simulink model "WDS_with_AttackDetection"  (R2021a)
settings: Solver=FixedStepDiscrete  StartTime=0.0  StopTime=T_final  FixedStep=T_sample  RelTol=1e-3
values from neighbouring files (symbols this model uses):
  A_bar_d = readmatrix('A_bar_d.csv')    [Run_model_with_attackDetection.m]
  attack_tank_full = zeros(size(attack_tank,1),n_meas)    [Run_results.m]    (also in Run_results_new.m; time_domain_sim.m)
  b1_1 = readmatrix(append(datapath,'MLP1\b1.csv'))    [Run_model_with_attackDetection.m]
  b1_2 = readmatrix(append(datapath,'MLP2\b1.csv'))    [Run_model_with_attackDetection.m]
  b2_1 = readmatrix(append(datapath,'MLP1\b2.csv'))    [Run_model_with_attackDetection.m]
  b2_2 = readmatrix(append(datapath,'MLP2\b2.csv'))    [Run_model_with_attackDetection.m]
  b3_1 = readmatrix(append(datapath,'MLP1\b3.csv'))    [Run_model_with_attackDetection.m]
  b3_2 = readmatrix(append(datapath,'MLP2\b3.csv'))    [Run_model_with_attackDetection.m]
  b4_1 = readmatrix(append(datapath,'MLP1\b4.csv'))    [Run_model_with_attackDetection.m]
  b4_2 = readmatrix(append(datapath,'MLP2\b4.csv'))    [Run_model_with_attackDetection.m]
  B_bar_d = readmatrix('B_bar_d.csv')    [Run_model_with_attackDetection.m]
  C_obsv_d = readmatrix('C_obsv_d.csv')    [Run_model_with_attackDetection.m]
  Cm = ones(1,n_states)    [Run_model_with_attackDetection.m]
  D_obsv_d = readmatrix('D_obsv_d.csv')    [Run_model_with_attackDetection.m]
  E0_full = zeros(T,n_meas)    [Run_results.m]    (also in Run_results_new.m; time_domain_sim.m)
  eta = 0.7    [Run_model_with_attackDetection.m]
  H0_perp_full = eye(size(H0_full,1)) - H0_full*H0_full_pinv    [Run_model_with_attackDetection.m]
  I_attack_local = I_attack(1:n_attack)    [Run_results.m]    (also in Run_results_new.m; time_domain_sim.m)
  K = place(A_bar_d,B_bar_d,Pc)    [Run_model_with_attackDetection.m]
  k0 = 42    [Run_model_with_attackDetection.m]
  Lu = F-A_bar_d.'*H0_full_pinv*H1_full    [Run_model_with_attackDetection.m]
  Ly = A_bar_d.'*H0_full_pinv    [Run_model_with_attackDetection.m]
  M1 = readmatrix('M1.csv')    [Run_model_with_attackDetection.m]
  M2 = readmatrix('M2.csv')    [Run_model_with_attackDetection.m]
  n_meas = size(C_obsv_d,1)    [Run_model_with_attackDetection.m]
  offset = -inv(B_bar_d)*(A_bar_d-eye(n_states))*xd    [Run_model_with_attackDetection.m]
  p_MLP1 = load('P1.mat').P1    [Run_model_with_attackDetection.m]
  p_MLP2 = load('P2.mat').P2    [Run_model_with_attackDetection.m]
  Q0 = ones(n_meas,T)    [Run_model_with_attackDetection.m]
  T = 8    [Run_model_with_attackDetection.m]    (also in align_attack_dataset.m)
  T_sample = 0.01    [Run_model_with_attackDetection.m]
  T_start_attack = 0.1*T_final    (= 0.8)    [Run_model_with_attackDetection.m]
  T_start_detect = T_start_attack+T*T_sample    (= 0.88)    [Run_model_with_attackDetection.m]
  tau2 = readmatrix('tau2.csv')    [Run_model_with_attackDetection.m]
  U0 = zeros(n_int,T+1)    [Run_model_with_attackDetection.m]
  w1_1 = readmatrix(append(datapath,'\MLP1\w1.csv'))    [Run_model_with_attackDetection.m]
  w1_2 = readmatrix(append(datapath,'\MLP2\w1.csv'))    [Run_model_with_attackDetection.m]
  w2_1 = readmatrix(append(datapath,'MLP1\w2.csv'))    [Run_model_with_attackDetection.m]
  w2_2 = readmatrix(append(datapath,'MLP2\w2.csv'))    [Run_model_with_attackDetection.m]
  w3_1 = readmatrix(append(datapath,'MLP1\w3.csv'))    [Run_model_with_attackDetection.m]
  w3_2 = readmatrix(append(datapath,'MLP2\w3.csv'))    [Run_model_with_attackDetection.m]
  w4_1 = readmatrix(append(datapath,'MLP1\w4.csv'))    [Run_model_with_attackDetection.m]
  w4_2 = readmatrix(append(datapath,'MLP2\w4.csv'))    [Run_model_with_attackDetection.m]
  x0 = 0.3+ 0.2*rand(n_states,1)    [Run_model_with_attackDetection.m]
  xd = 0.5*ones(n_states,1)    [Run_model_with_attackDetection.m]
  Y0 = zeros(n_meas,T)    [Run_model_with_attackDetection.m]
undefined symbols (not defined in the file or in its folder): F, H0_full, H1_full, n_int, n_states, T_start_opt
libraries: simulink x15
(part 2 of 2)

== matlab function WDS_with_AttackDetection/False Data Injection Attacks3/sample_based Moving-horizon FDIA ==
  data: E output; e output double; et input; attack_tank_full parameter; M1 parameter; M2 parameter; tau2 parameter; T parameter
function [E,e] = fcn(et, attack_tank_full, M1, M2,tau2,T)
%% function [E,e] = fcn(et, attack_tank_full, M1, M2,tau2)
% sample-based moving horizon FDIA
% optimization problem or returns zeros if infeasible:
%         Maximize: ||M1*[e_history; e_i]||_2 
%         Subject to: ||M2*[e_history; e_i||_2 <= tau
%                      e_i \in e_data
% Inputs: 
%         - et [n_meas-by-T]         : cahce
%         - attack_tank_full [N_data-by-n_meas]: tank of pre-generated attacks
%         - M1 [n_m1-by-(T*n_meas)]  : Attack impact operator
%         - M2 [n_m2-by-(T*n_meas)]  : Detection residual operator
%         - tau2 [scalar]            : Detection threshold
% Output:
%         - E [n_meas-by-T] : cahce
%         - e [n_meas-by-1] : current-time-step attack
%
% Yu zheng, RASLab, FAMU-FSU College of Engineering, Tallahassee, 2021, Aug.



%% get T-1 attacks history
E_history = et(:,2:end).';  % [n_meas-by-(T-1)]
e_history = E_history(:);  % [n_meas*(T-1)-by-1]

%% get current attack
e = getCurrentAttack(e_history,M1,M2,tau2,attack_tank_full,T);

%% update cache E (save T recent attacks)
et(:,1:end-1) = et(:,2:end);
et(:,end) = e;
E = et;

== matlab function WDS_with_AttackDetection/Tapped Delay7/tapped_delay1 ==
  data: t input; q input; qt input; Q output; n_meas parameter; T_start_detect parameter; T parameter
function Q  = fcn(t, q,qt,n_meas,T_start_detect, T)
%% tapped_delay_array
% shift columns from tapped matrix to the left and appends most recent
% vector to the last column
% %%% input
% ut(:,1:end-1) = ut(:,2:end);
% ut(:,end) = u;
% U = ut;
% %%% output
% yt(:,1:end-1) = yt(:,2:end);
% yt(:,end) = y;
% Y = yt;
%%% pruning support
Q = ones(n_meas,T);
if t>T_start_detect
    qt(:,1:end-1) = qt(:,2:end);
    qt(:,end) = q;
    Q = qt;
end
end

== matlab function WDS_with_AttackDetection/Water-tank system ==
  data: x input; x_next output; u input; v input; y output; A_bar_d parameter; C_obsv_d parameter; B_bar_d parameter; D_obsv_d parameter; yc output; Cm parameter
function [x_next,y,yc] = fcn(x,u,v,A_bar_d,C_obsv_d,B_bar_d,D_obsv_d,Cm)
% Discrete state-space model for system

x_next = A_bar_d*x + B_bar_d*u - v;

y = C_obsv_d*x + D_obsv_d*u;

% critical measurements
yc = Cm*x;

== matlab function WDS_with_AttackDetection/Tapped Delay2/tapped_delay ==
  data: u input; U output; ut input; y input; yt input; Y output
function [U,Y] = fcn(u,ut,y,yt)
%% tapped_delay_array
% shift columns from tapped matrix to the left and appends most recent
% vector to the last column
%%% input
ut(:,1:end-1) = ut(:,2:end);
ut(:,end) = u;
U = ut;
%%% output
yt(:,1:end-1) = yt(:,2:end);
yt(:,end) = y;
Y = yt;

== matlab function WDS_with_AttackDetection/Receding L2 Observer1/ResilientOptimzer ==
  data: prune_mask_out output; x_next output; U input; Y input; Q input; n_int parameter; T parameter; H0_perp_full parameter; H0_full parameter; r output; n_states parameter; H1_full parameter; F parameter; A_bar_d parameter
function [prune_mask_out,x_next,r]  = fcn(U,Y,Q,n_int,T,H0_perp_full,H0_full, n_states, H1_full,F, A_bar_d)

u_local = zeros(n_int,T+1-1);
u_local(:,:) = U(:,1:end-1);
% vectorized
u = u_local(:);
y = Y(:);
q_eta_hat = Q(:);

%% pruning
prune_mask_out = sum(q_eta_hat>0.5);   % mask for safe nodes
prune_mask = find(q_eta_hat>0.5); %find(q_eta_hat>0.5); % true(size(q_eta_hat,1),1);

H0_eta = H0_full(prune_mask,:);
H1_eta = H1_full(prune_mask,:);

H0_eta_pinv = pinv(H0_eta,0.001);
Ly = A_bar_d.'*H0_eta_pinv;
Lu = F-A_bar_d.'*H0_eta_pinv*H1_eta;

x_next = zeros(n_states,1);
x_next(:) = Ly*y(prune_mask) + Lu*u;

r = H0_perp_full*(y-H1_full*u);

== matlab function WDS_with_AttackDetection/Water-tank system_attack ==
  data: x input; x_next output; u input; v input; y output; A_bar_d parameter; C_obsv_d parameter; B_bar_d parameter; D_obsv_d parameter; yc output; Cm parameter
function [x_next,y,yc] = fcn(x,u,v,A_bar_d,C_obsv_d,B_bar_d,D_obsv_d,Cm)
% Discrete state-space model for system

x_next = A_bar_d*x + B_bar_d*u - v;

y = C_obsv_d*x + D_obsv_d*u;

% critical measurements
yc = Cm*x;

== matlab function WDS_with_AttackDetection/Random Demand/ random demand ==
  data: v output; n_states parameter
function v = fcn(n_states)

v = 0.3*rand(n_states,1);
